simulink model "simulation"  (R2013b)
settings: Solver=ode45  StartTime=0.0  StopTime=2000  RelTol=1e-3
values from neighbouring files (symbols this model uses):
  delta = .5    (= 0.5)    [simulation_init.m]
  Fmax = 1000    [simulation_init.m]
  Fmin = -750    [simulation_init.m]
  J = I_z - N    (= 2752.5)    [simulation_init.m]
  k_r = .5    (= 0.5)    [simulation_init.m]
  k_u = .5    (= 0.5)    [simulation_init.m]
  k_xi = 1    [simulation_init.m]
  kx = .3    (= 0.3)    [simulation_init.m]
  ky = .15    (= 0.15)    [simulation_init.m]
  kz = 1.5    [simulation_init.m]
  l = 1    [simulation_init.m]
  m_u = m - Xm_u    (= 4287.13636)    [simulation_init.m]
  m_uv = Xm_v - Xm_u    (= -28.713636)    [simulation_init.m]
  m_v = m - Xm_v    (= 4315.849996)    [simulation_init.m]
  n = 4    [simulation_init.m]
  noiseon = 1    [simulation_init.m]
  npsi = 0.00005    (= 5e-05)    [simulation_init.m]
  npsi_c = 0*.00005    (= 0)    [simulation_init.m]
  Nr = -110    [simulation_init.m]
  nr = 0.005    [simulation_init.m]
  Nrr = -555    [simulation_init.m]
  nsonar = .1    (= 0.1)    [simulation_init.m]
  nu = .05    (= 0.05)    [simulation_init.m]
  nv = 0.005    [simulation_init.m]
  nVc = 0*.005    (= 0)    [simulation_init.m]
  P01 = [20   20]    [simulation_init.m]
  P02 = [40   00]    [simulation_init.m]
  P03 = [20  -20]    [simulation_init.m]
  P04 = [150 40]    [simulation_init.m]
  psi01 = 0*pi/180    (= 0)    [simulation_init.m]
  psi02 = 0*pi/180    (= 0)    [simulation_init.m]
  psi03 = 0*pi/180    (= 0)    [simulation_init.m]
  psi_c = 45*pi/180    (= 0.785398163397)    [simulation_init.m]
  Q1 = diag([nu nv npsi])    [simulation_init.m]
  Q2 = diag([nu nv npsi])    [simulation_init.m]
  Q3 = diag([nu nv npsi])    [simulation_init.m]
  Sigma01 = 15*eye(3)    [simulation_init.m]
  Sigma02 = Sigma01    [simulation_init.m]
  Sigma03 = Sigma01    [simulation_init.m]
  State_est01 = [P01+[sN(1),sN(2)] psi01]    [simulation_init.m]
  State_est02 = [P02+[sN(3),sN(4)] psi02]    [simulation_init.m]
  State_est03 = [P03+[sN(5),sN(6)] psi03]    [simulation_init.m]
  T_bc = 1    [simulation_init.m]
  T_est = .1    (= 0.1)    [simulation_init.m]
  Vc = .3    (= 0.3)    [simulation_init.m]
  Xu = -360    [simulation_init.m]
  Xuu = -805    [simulation_init.m]
  Yv = -420    [simulation_init.m]
  Yvv = -1930    [simulation_init.m]
undefined symbols (not defined in the file or in its folder): Pathdata
libraries: simulink x22
(part 1 of 2)
settings Model: Creator=Andreas  LastModifiedBy=Andreas

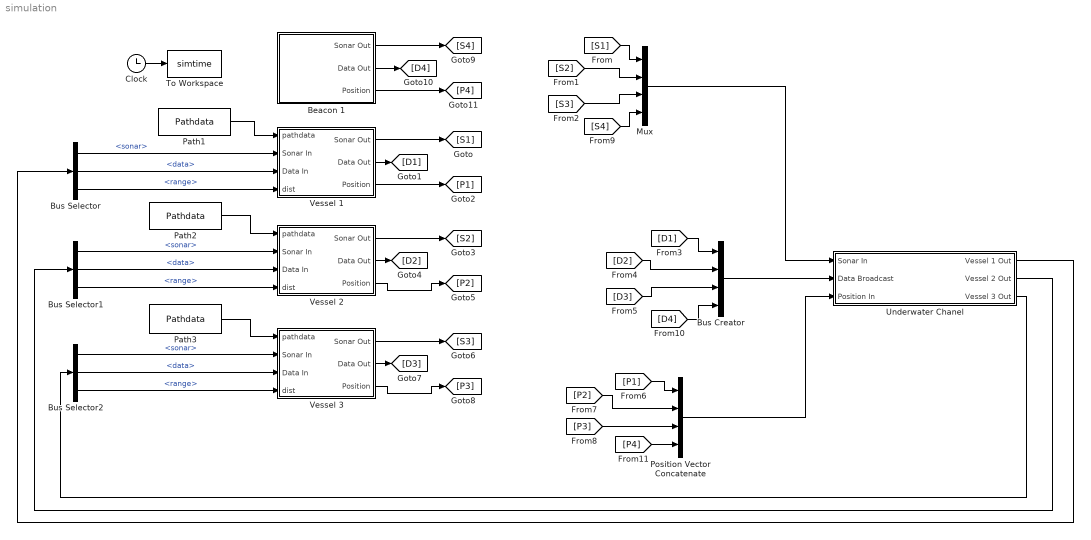
== system simulation ==
  Beacon 1 : Subsystem  mask{i=4}
      mask prompts: i "id"
  Bus Creator : BusCreator
  Bus Selector : BusSelector  OutputSignals=sonar,data,range
  Bus Selector1 : BusSelector  OutputSignals=sonar,data,range
  Bus Selector2 : BusSelector  OutputSignals=sonar,data,range
  Clock : Clock
  Mux : Mux
  Path1 : Constant  Value=Pathdata
  Path2 : Constant  Value=Pathdata
  Path3 : Constant  Value=Pathdata
  Position Vector Concatenate : Concatenate  NumInputs=4  Mode=Multidimensional array  ConcatenateDimension=2
  To Workspace : ToWorkspace  VariableName=simtime  SampleTime=-1
  Underwater Chanel : Subsystem
  Vessel 1 : Subsystem  mask{i=1}
      mask prompts: i "id"
      mask init:
      | Maskinit
  Vessel 2 : Subsystem  mask{i=2}
      mask prompts: i "id"
      mask init:
      | Maskinit
  Vessel 3 : Subsystem  mask{i=3}
      mask prompts: i "id"
      mask init:
      | Maskinit
  wires:
  Underwater Chanel/1(Vessel 1 Out) -> Bus Selector/1
  Underwater Chanel/2(Vessel 2 Out) -> Bus Selector1/1
  Underwater Chanel/3(Vessel 3 Out) -> Bus Selector2/1
  [S1] -> Mux/1
  [S3] -> Mux/3
  [D1] -> Bus Creator/1
  [D2] -> Bus Creator/2
  [D3] -> Bus Creator/3
  [P2] -> Position Vector Concatenate/2
  [P1] -> Position Vector Concatenate/1
  [P3] -> Position Vector Concatenate/3
  Vessel 1/1(Sonar Out) -> [S1]
  Vessel 1/2(Data Out) -> [D1]
  Vessel 1/3(Position) -> [P1]
  Vessel 2/1(Sonar Out) -> [S2]
  Vessel 2/2(Data Out) -> [D2]
  Vessel 2/3(Position) -> [P2]
  Vessel 3/1(Sonar Out) -> [S3]
  Vessel 3/2(Data Out) -> [D3]
  Vessel 3/3(Position) -> [P3]
  Position Vector Concatenate/1 -> Underwater Chanel/3(Position In)
  [S2] -> Mux/2
  Path1/1 -> Vessel 1/1(pathdata)
  Path2/1 -> Vessel 2/1(pathdata)
  Path3/1 -> Vessel 3/1(pathdata)
  Clock/1 -> To Workspace/1
  Beacon 1/1(Sonar Out) -> [S4]
  Beacon 1/2(Data Out) -> [D4]
  Beacon 1/3(Position) -> [P4]
  [S4] -> Mux/4
  [D4] -> Bus Creator/4
  [P4] -> Position Vector Concatenate/4
  Bus Selector/2 -> Vessel 1/3(Data In)  "<data>"
  Bus Selector/1 -> Vessel 1/2(Sonar In)  "<sonar>"
  Bus Selector/3 -> Vessel 1/4(dist)  "<range>"
  Bus Selector2/1 -> Vessel 3/2(Sonar In)  "<sonar>"
  Bus Selector2/3 -> Vessel 3/4(dist)  "<range>"
  Bus Selector2/2 -> Vessel 3/3(Data In)  "<data>"
  Bus Selector1/3 -> Vessel 2/4(dist)  "<range>"
  Bus Selector1/2 -> Vessel 2/3(Data In)  "<data>"
  Bus Selector1/1 -> Vessel 2/2(Sonar In)  "<sonar>"
  Mux/1 -> Underwater Chanel/1(Sonar In)
  Bus Creator/1 -> Underwater Chanel/2(Data Broadcast)

== system simulation/Beacon 1 ==
  Constant : Constant
  Cov : Constant  Value=0.0001*[1 0 0 1]
  Fixed Position : Constant  Value=[P04 0]
  Fixed Position2 : Constant  Value=P04
  JLaw : simulink/Sources/Repeating Sequence Stair  OutValues=TrsmtLaw.'  tsamp=T_bc  OutMin=[]  OutMax=[]  OutDataTypeStr=double  OutputDataTypeScalingMode=double  OutDataType=fixdt(0,8)  ConRadixGroup=Best Precision: Vector-wise  OutScaling=2^-12
  Transmitter : Subsystem
  data_out : ToWorkspace  VariableName=data_out4  SampleTime=-1
  sonar_out : ToWorkspace  VariableName=sonar_out4  SampleTime=-1
  Sonar Out : Outport
  Data Out : Outport  Port=2
  Position : Outport  Port=3
  wires:
  Constant/1 -> Transmitter/3(gamma_i1)
  JLaw/1 -> Transmitter/1(j1)
  Fixed Position/1 -> Position/1
  Transmitter/1(Sonar Out) -> sonar_out/1, Sonar Out/1
  Transmitter/2(Data Out) -> Data Out/1, data_out/1
  Cov/1 -> Transmitter/4(cov1)
  Fixed Position2/1 -> Transmitter/2(state1)

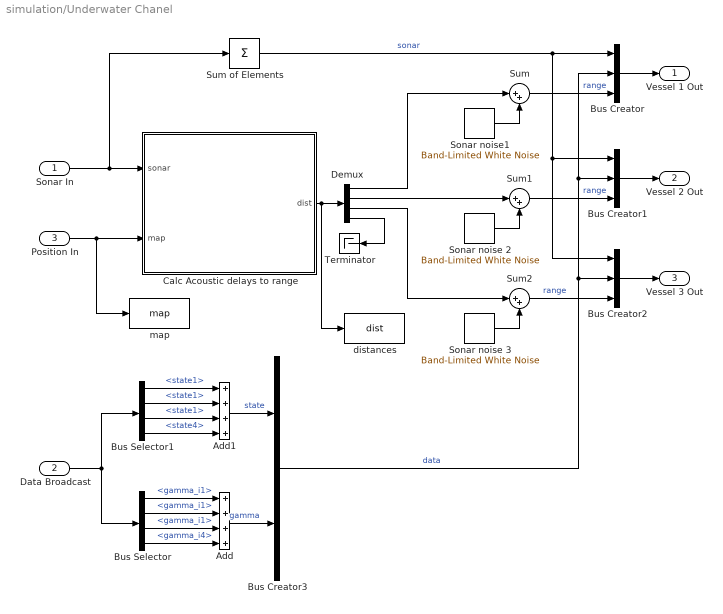
== system simulation/Underwater Chanel ==
  Sonar In : Inport
  Data Broadcast : Inport  Port=2
  Position In : Inport  Port=3
  Add : Sum  Inputs=++++
  Add1 : Sum  Inputs=++++
  Bus Creator : BusCreator  Inputs=3
  Bus Creator1 : BusCreator  Inputs=3
  Bus Creator2 : BusCreator  Inputs=3
  Bus Creator3 : BusCreator  Inputs=2
  Bus Selector : BusSelector  OutputSignals=signal1.gamma_i1,signal2.gamma_i1,signal3.gamma_i1,signal4.gamma_i4
  Bus Selector1 : BusSelector  OutputSignals=signal1.state1,signal2.state1,signal3.state1,signal4.state4
  Calc Acoustic delays to range : MATLAB Function  TreatAsAtomicUnit=on
  Demux : Demux
  Sonar noise 2 : simulink/Sources/Band-Limited White Noise  Cov=noiseon*nsonar*0.1  Ts=0.1  seed=535
  Sonar noise 3 : simulink/Sources/Band-Limited White Noise  Cov=noiseon*nsonar*0.1  Ts=0.1  seed=24
  Sonar noise1 : simulink/Sources/Band-Limited White Noise  Cov=noiseon*nsonar*0.1  Ts=0.1  seed=[253]
  Sum : Sum  Inputs=|++
  Sum of Elements : Sum  Inputs=+
  Sum1 : Sum  Inputs=|++
  Sum2 : Sum  Inputs=|++
  Terminator : Terminator
  distances : ToWorkspace  VariableName=dist  SampleTime=-1
  map : ToWorkspace  VariableName=map  SampleTime=-1
  Vessel 1 Out : Outport
  Vessel 2 Out : Outport  Port=2
  Vessel 3 Out : Outport  Port=3
  wires:
  Position In/1 -> map/1, Calc Acoustic delays to range/2(map)
  Bus Creator/1 -> Vessel 1 Out/1
  Bus Creator2/1 -> Vessel 3 Out/1
  Calc Acoustic delays to range/1(dist) -> distances/1, Demux/1
  Sonar In/1 -> Sum of Elements/1, Calc Acoustic delays to range/1(sonar)
  Bus Creator1/1 -> Vessel 2 Out/1
  Data Broadcast/1 -> Bus Selector1/1, Bus Selector/1
  Sum of Elements/1 -> Bus Creator/1, Bus Creator2/1, Bus Creator1/1  "sonar"
  Demux/4 -> Terminator/1
  Sum/1 -> Bus Creator/3  "range"
  Demux/1 -> Sum/1
  Sonar noise1/1 -> Sum/2
  Sonar noise 2/1 -> Sum1/2
  Demux/2 -> Sum1/1
  Sum1/1 -> Bus Creator1/3  "range"
  Sonar noise 3/1 -> Sum2/2
  Demux/3 -> Sum2/1
  Sum2/1 -> Bus Creator2/3  "range"
  Bus Selector/2 -> Add/2  "<gamma_i1>"
  Bus Selector/1 -> Add/1  "<gamma_i1>"
  Bus Selector/3 -> Add/3  "<gamma_i1>"
  Bus Selector1/3 -> Add1/3  "<state1>"
  Bus Selector1/1 -> Add1/1  "<state1>"
  Bus Selector1/4 -> Add1/4  "<state4>"
  Bus Selector1/2 -> Add1/2  "<state1>"
  Add1/1 -> Bus Creator3/1  "state"
  Add/1 -> Bus Creator3/2  "gamma"
  Bus Creator3/1 -> Bus Creator2/2, Bus Creator1/2, Bus Creator/2  "data"
  Bus Selector/4 -> Add/4  "<gamma_i4>"

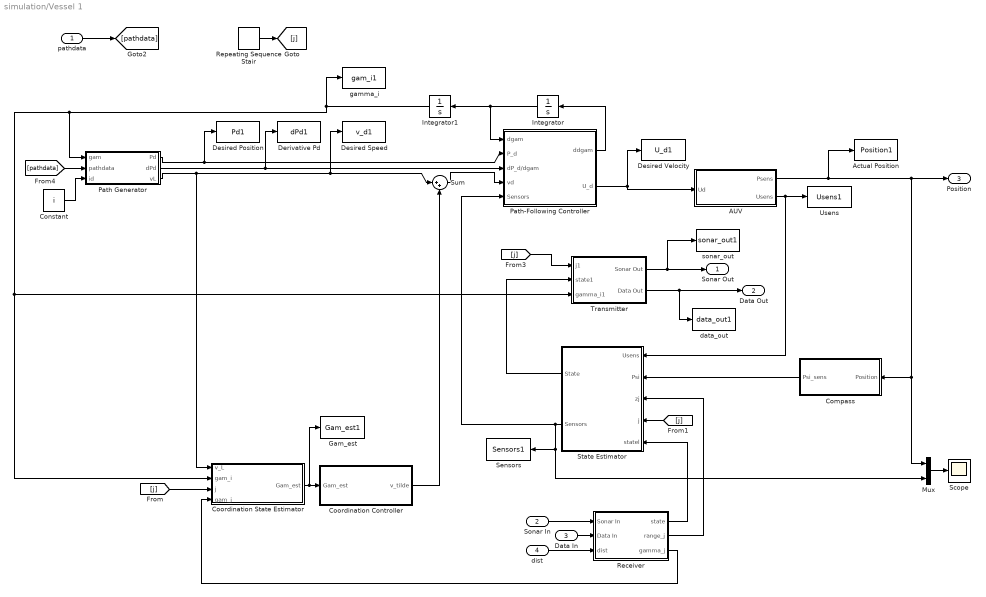
== system simulation/Vessel 1 ==
  pathdata : Inport
  Sonar In : Inport  Port=2
  Data In : Inport  Port=3
  dist : Inport  Port=4
  AUV : Subsystem
  Actual Position : ToWorkspace  VariableName=Position1  SampleTime=-1
  Compass : Subsystem
  Constant : Constant  Value=i
  Coordination Controller : MATLAB Function  TreatAsAtomicUnit=on
  Coordination State Estimator : Subsystem
  Derivative Pd : ToWorkspace  VariableName=dPd1  SampleTime=-1
  Desired Position : ToWorkspace  VariableName=Pd1  SampleTime=-1
  Desired Speed : ToWorkspace  VariableName=v_d1  SampleTime=-1
  Desired Velocity : ToWorkspace  VariableName=U_d1  SampleTime=-1
  Gam_est : ToWorkspace  VariableName=Gam_est1  SampleTime=-1
  Integrator : Integrator
  Integrator1 : Integrator
  Mux : Mux  Inputs=2
  Path Generator : Subsystem
  Path-Following Controller : Subsystem
  Receiver : Subsystem
  Repeating Sequence Stair : simulink/Sources/Repeating Sequence Stair  OutValues=TrsmtLaw.'  tsamp=T_bc  OutMin=[]  OutMax=[]  OutDataTypeStr=double  OutputDataTypeScalingMode=double  OutDataType=fixdt(0,8)  ConRadixGroup=Best Precision: Vector-wise  OutScaling=2^-12
  Scope : Scope
      settings: YMin=-25  YMax=275
  Sensors : ToWorkspace  VariableName=Sensors1  SampleTime=-1
  State Estimator : Subsystem
  Sum : Sum  Inputs=|++
  Transmitter : Subsystem
  Usens : ToWorkspace  VariableName=Usens1  SampleTime=-1
  data_out : ToWorkspace  VariableName=data_out1  SampleTime=-1
  gamma_i : ToWorkspace  VariableName=gam_i1  SampleTime=-1
  sonar_out : ToWorkspace  VariableName=sonar_out1  SampleTime=-1
  Sonar Out : Outport
  Data Out : Outport  Port=2
  Position : Outport  Port=3
  wires:
  Sonar In/1 -> Receiver/1(Sonar In)
  Data In/1 -> Receiver/2(Data In)
  Integrator1/1 -> gamma_i/1, Path Generator/1(gam), Transmitter/3(gamma_i1), Coordination State Estimator/2(gam_i)
  Path Generator/3(vL) -> Coordination State Estimator/1(v_L), Desired Speed/1, Sum/1
  Coordination Controller/1(v_tilde) -> Sum/2
  Sum/1 -> Path-Following Controller/4(vd)
  Transmitter/1(Sonar Out) -> sonar_out/1, Sonar Out/1
  Transmitter/2(Data Out) -> data_out/1, Data Out/1
  Receiver/3(gamma_j) -> Coordination State Estimator/4(gam_j)
  Path Generator/1(Pd) -> Desired Position/1, Path-Following Controller/2(P_d)
  Path-Following Controller/1(ddgam) -> Integrator/1
  Integrator/1 -> Integrator1/1, Path-Following Controller/1(dgam)
  Path-Following Controller/2(U_d) -> AUV/1(Ud), Desired Velocity/1
  AUV/2(Usens) -> Usens/1, State Estimator/1(Usens)
  AUV/1(Psens) -> Mux/1, Compass/1(Position), Position/1, Actual Position/1
  Coordination State Estimator/1(Gam_est) -> Gam_est/1, Coordination Controller/1(Gam_est)
  Path Generator/2(dPd) -> Path-Following Controller/3(dP_d/dgam), Derivative Pd/1
  Repeating Sequence Stair/1 -> [j]
  [j] -> Coordination State Estimator/3(j)
  dist/1 -> Receiver/3(dist)
  Constant/1 -> Path Generator/3(id)
  pathdata/1 -> [pathdata]
  [pathdata] -> Path Generator/2(pathdata)
  State Estimator/2(Sensors) -> Sensors/1, Mux/2, Path-Following Controller/5(Sensors)
  [j] -> Transmitter/1(j1)
  [j] -> State Estimator/4(j)
  State Estimator/1("State ") -> Transmitter/2(state1)
  Receiver/1(state) -> State Estimator/5(statel)
  Mux/1 -> Scope/1
  Compass/1(Psi_sens) -> State Estimator/2(Psi)
  Receiver/2(range_j) -> State Estimator/3(zj)

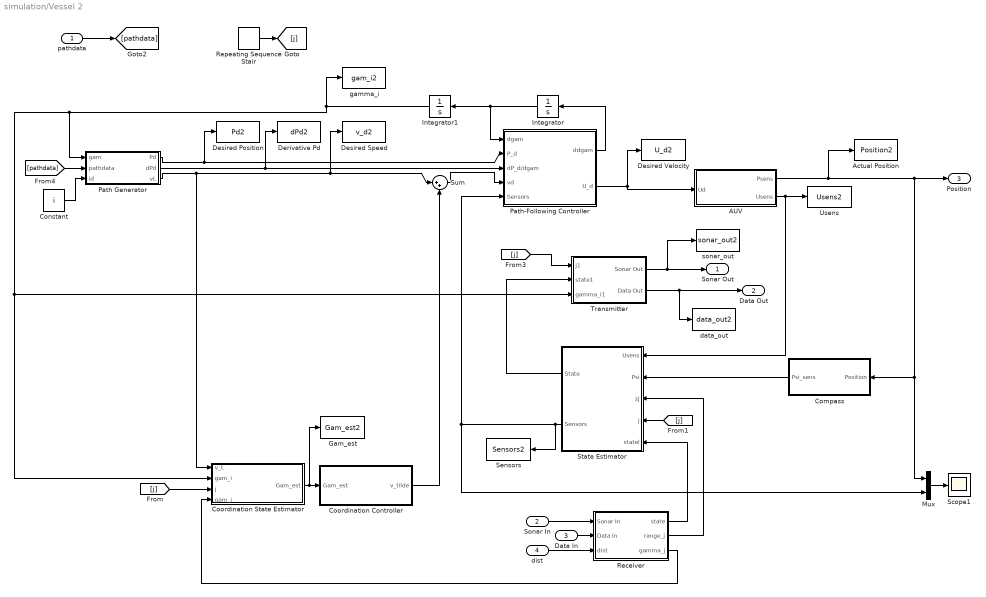
== system simulation/Vessel 2 ==
  pathdata : Inport
  Sonar In : Inport  Port=2
  Data In : Inport  Port=3
  dist : Inport  Port=4
  AUV : Subsystem
  Actual Position : ToWorkspace  VariableName=Position2  SampleTime=-1
  Compass : Subsystem
  Constant : Constant  Value=i
  Coordination Controller : MATLAB Function  TreatAsAtomicUnit=on
  Coordination State Estimator : Subsystem
  Derivative Pd : ToWorkspace  VariableName=dPd2  SampleTime=-1
  Desired Position : ToWorkspace  VariableName=Pd2  SampleTime=-1
  Desired Speed : ToWorkspace  VariableName=v_d2  SampleTime=-1
  Desired Velocity : ToWorkspace  VariableName=U_d2  SampleTime=-1
  Gam_est : ToWorkspace  VariableName=Gam_est2  SampleTime=-1
  Integrator : Integrator
  Integrator1 : Integrator
  Mux : Mux  Inputs=2
  Path Generator : Subsystem
  Path-Following Controller : Subsystem
  Receiver : Subsystem
  Repeating Sequence Stair : simulink/Sources/Repeating Sequence Stair  OutValues=TrsmtLaw.'  tsamp=T_bc  OutMin=[]  OutMax=[]  OutDataTypeStr=double  OutputDataTypeScalingMode=double  OutDataType=fixdt(0,8)  ConRadixGroup=Best Precision: Vector-wise  OutScaling=2^-12
  Scope1 : Scope
      settings: YMin=-25  YMax=275
  Sensors : ToWorkspace  VariableName=Sensors2  SampleTime=-1
  State Estimator : Subsystem
  Sum : Sum  Inputs=|++
  Transmitter : Subsystem
  Usens : ToWorkspace  VariableName=Usens2  SampleTime=-1
  data_out : ToWorkspace  VariableName=data_out2  SampleTime=-1
  gamma_i : ToWorkspace  VariableName=gam_i2  SampleTime=-1
  sonar_out : ToWorkspace  VariableName=sonar_out2  SampleTime=-1
  Sonar Out : Outport
  Data Out : Outport  Port=2
  Position : Outport  Port=3
  wires:
  Receiver/1(state) -> State Estimator/5(statel)
  State Estimator/1("State ") -> Transmitter/2(state1)
  [j] -> State Estimator/4(j)
  [j] -> Transmitter/1(j1)
  [pathdata] -> Path Generator/2(pathdata)
  pathdata/1 -> [pathdata]
  Constant/1 -> Path Generator/3(id)
  dist/1 -> Receiver/3(dist)
  [j] -> Coordination State Estimator/3(j)
  Repeating Sequence Stair/1 -> [j]
  Path Generator/2(dPd) -> Derivative Pd/1, Path-Following Controller/3(dP_d/dgam)
  Coordination State Estimator/1(Gam_est) -> Coordination Controller/1(Gam_est), Gam_est/1
  AUV/2(Usens) -> State Estimator/1(Usens), Usens/1
  Path-Following Controller/2(U_d) -> Desired Velocity/1, AUV/1(Ud)
  Integrator/1 -> Path-Following Controller/1(dgam), Integrator1/1
  Path-Following Controller/1(ddgam) -> Integrator/1
  Path Generator/1(Pd) -> Path-Following Controller/2(P_d), Desired Position/1
  Receiver/3(gamma_j) -> Coordination State Estimator/4(gam_j)
  Transmitter/2(Data Out) -> Data Out/1, data_out/1
  Transmitter/1(Sonar Out) -> Sonar Out/1, sonar_out/1
  Sum/1 -> Path-Following Controller/4(vd)
  Coordination Controller/1(v_tilde) -> Sum/2
  Path Generator/3(vL) -> Sum/1, Desired Speed/1, Coordination State Estimator/1(v_L)
  Integrator1/1 -> Coordination State Estimator/2(gam_i), Transmitter/3(gamma_i1), Path Generator/1(gam), gamma_i/1
  Data In/1 -> Receiver/2(Data In)
  Sonar In/1 -> Receiver/1(Sonar In)
  AUV/1(Psens) -> Actual Position/1, Compass/1(Position), Mux/1, Position/1
  State Estimator/2(Sensors) -> Path-Following Controller/5(Sensors), Mux/2, Sensors/1
  Mux/1 -> Scope1/1
  Compass/1(Psi_sens) -> State Estimator/2(Psi)
  Receiver/2(range_j) -> State Estimator/3(zj)

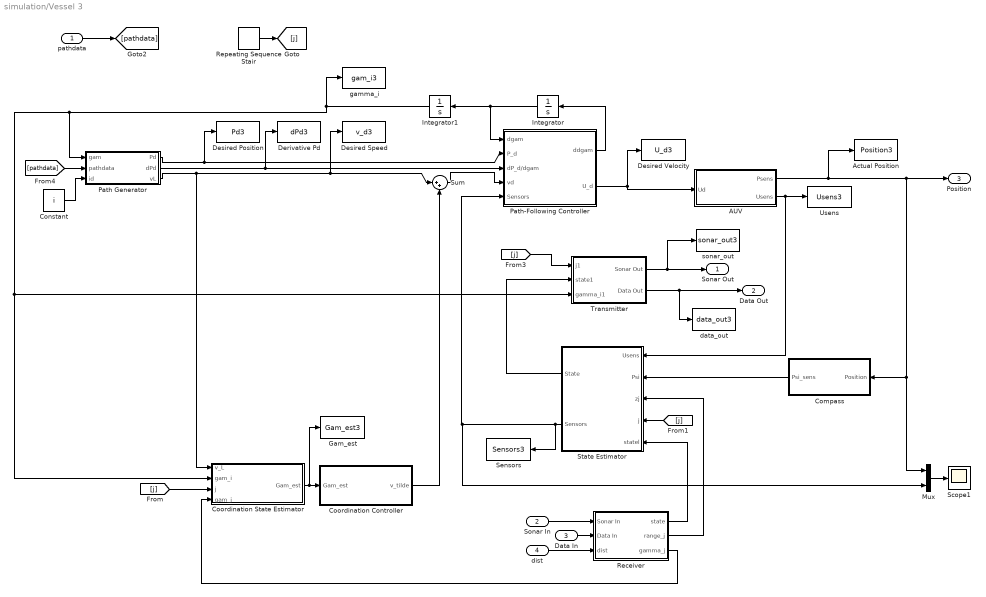
== system simulation/Vessel 3 ==
  pathdata : Inport
  Sonar In : Inport  Port=2
  Data In : Inport  Port=3
  dist : Inport  Port=4
  AUV : Subsystem
  Actual Position : ToWorkspace  VariableName=Position3  SampleTime=-1
  Compass : Subsystem
  Constant : Constant  Value=i
  Coordination Controller : MATLAB Function  TreatAsAtomicUnit=on
  Coordination State Estimator : Subsystem
  Derivative Pd : ToWorkspace  VariableName=dPd3  SampleTime=-1
  Desired Position : ToWorkspace  VariableName=Pd3  SampleTime=-1
  Desired Speed : ToWorkspace  VariableName=v_d3  SampleTime=-1
  Desired Velocity : ToWorkspace  VariableName=U_d3  SampleTime=-1
  Gam_est : ToWorkspace  VariableName=Gam_est3  SampleTime=-1
  Integrator : Integrator
  Integrator1 : Integrator
  Mux : Mux  Inputs=2
  Path Generator : Subsystem
  Path-Following Controller : Subsystem
  Receiver : Subsystem
  Repeating Sequence Stair : simulink/Sources/Repeating Sequence Stair  OutValues=TrsmtLaw.'  tsamp=T_bc  OutMin=[]  OutMax=[]  OutDataTypeStr=double  OutputDataTypeScalingMode=double  OutDataType=fixdt(0,8)  ConRadixGroup=Best Precision: Vector-wise  OutScaling=2^-12
  Scope1 : Scope
      settings: YMin=-10  YMax=130  SaveName=ScopeData2
  Sensors : ToWorkspace  VariableName=Sensors3  SampleTime=-1
  State Estimator : Subsystem
  Sum : Sum  Inputs=|++
  Transmitter : Subsystem
  Usens : ToWorkspace  VariableName=Usens3  SampleTime=-1
  data_out : ToWorkspace  VariableName=data_out3  SampleTime=-1
  gamma_i : ToWorkspace  VariableName=gam_i3  SampleTime=-1
  sonar_out : ToWorkspace  VariableName=sonar_out3  SampleTime=-1
  Sonar Out : Outport
  Data Out : Outport  Port=2
  Position : Outport  Port=3
  wires:
  Sonar In/1 -> Receiver/1(Sonar In)
  Data In/1 -> Receiver/2(Data In)
  Integrator1/1 -> gamma_i/1, Path Generator/1(gam), Transmitter/3(gamma_i1), Coordination State Estimator/2(gam_i)
  Path Generator/3(vL) -> Coordination State Estimator/1(v_L), Desired Speed/1, Sum/1
  Coordination Controller/1(v_tilde) -> Sum/2
  Sum/1 -> Path-Following Controller/4(vd)
  Transmitter/1(Sonar Out) -> sonar_out/1, Sonar Out/1
  Transmitter/2(Data Out) -> data_out/1, Data Out/1
  Receiver/3(gamma_j) -> Coordination State Estimator/4(gam_j)
  Path Generator/1(Pd) -> Desired Position/1, Path-Following Controller/2(P_d)
  Path-Following Controller/1(ddgam) -> Integrator/1
  Integrator/1 -> Integrator1/1, Path-Following Controller/1(dgam)
  Path-Following Controller/2(U_d) -> AUV/1(Ud), Desired Velocity/1
  AUV/2(Usens) -> Usens/1, State Estimator/1(Usens)
  Coordination State Estimator/1(Gam_est) -> Gam_est/1, Coordination Controller/1(Gam_est)
  Path Generator/2(dPd) -> Path-Following Controller/3(dP_d/dgam), Derivative Pd/1
  Repeating Sequence Stair/1 -> [j]
  [j] -> Coordination State Estimator/3(j)
  dist/1 -> Receiver/3(dist)
  Constant/1 -> Path Generator/3(id)
  pathdata/1 -> [pathdata]
  [pathdata] -> Path Generator/2(pathdata)
  [j] -> Transmitter/1(j1)
  [j] -> State Estimator/4(j)
  State Estimator/1("State ") -> Transmitter/2(state1)
  Receiver/1(state) -> State Estimator/5(statel)
  AUV/1(Psens) -> Position/1, Compass/1(Position), Mux/1, Actual Position/1
  State Estimator/2(Sensors) -> Sensors/1, Path-Following Controller/5(Sensors), Mux/2
  Mux/1 -> Scope1/1
  Compass/1(Psi_sens) -> State Estimator/2(Psi)
  Receiver/2(range_j) -> State Estimator/3(zj)

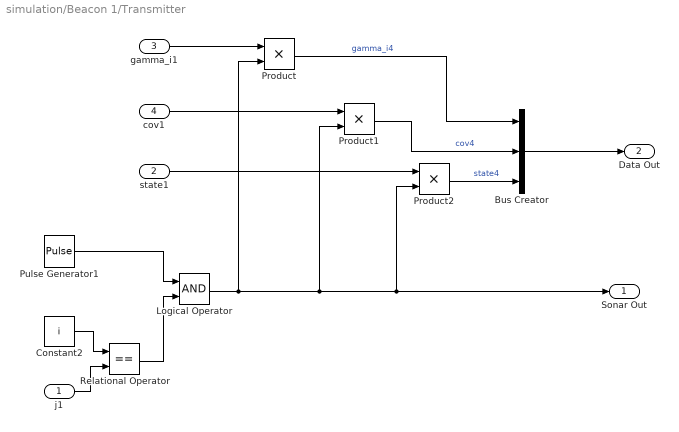
== system simulation/Beacon 1/Transmitter ==
  j1 : Inport
  state1 : Inport  Port=2
  gamma_i1 : Inport  Port=3
  cov1 : Inport  Port=4
  Bus Creator : BusCreator  Inputs=3
  Constant2 : Constant  Value=i
  Logical Operator : Logic  AllPortsSameDT=off  OutDataTypeStr=boolean
  Product : Product
  Product1 : Product
  Product2 : Product
  Pulse Generator1 : DiscretePulseGenerator  PulseType=Time based  Period=T_bc  PulseWidth=.001/( T_bc)*100
  Relational Operator : RelationalOperator  Operator===  OutDataTypeStr=boolean
  Sonar Out : Outport
  Data Out : Outport  Port=2
  wires:
  Pulse Generator1/1 -> Logical Operator/1
  j1/1 -> Relational Operator/2
  Constant2/1 -> Relational Operator/1
  Relational Operator/1 -> Logical Operator/2
  Logical Operator/1 -> Product/2, Product1/2, Product2/2, Sonar Out/1
  Bus Creator/1 -> Data Out/1
  gamma_i1/1 -> Product/1
  cov1/1 -> Product1/1
  state1/1 -> Product2/1
  Product/1 -> Bus Creator/1  "gamma_i4"
  Product1/1 -> Bus Creator/2  "cov4"
  Product2/1 -> Bus Creator/3  "state4"

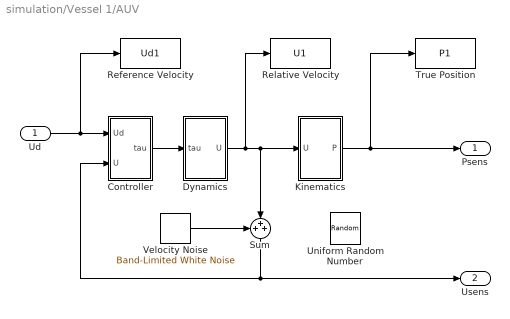
== system simulation/Vessel 1/AUV ==
  Ud : Inport
  Controller : Subsystem
  Dynamics : Subsystem
  Kinematics : Subsystem
  Reference Velocity : ToWorkspace  VariableName=Ud1  SampleTime=-1
  Relative Velocity : ToWorkspace  VariableName=U1  SampleTime=-1
  Sum : Sum  Inputs=+++
  True Position : ToWorkspace  VariableName=P1  SampleTime=-1
  Uniform Random Number : UniformRandomNumber  Minimum=-5*noiseon*[nu nv nr]  Maximum=5*noiseon*[nu nv nr]  Seed=[1627 9317 3723]  SampleTime=20
  Velocity Noise : simulink/Sources/Band-Limited White Noise  Cov=noiseon*[nu nv nr]*0.1  Ts=0.1  seed=[2334 8715 567]
  Psens : Outport
  Usens : Outport  Port=2
  wires:
  Dynamics/1(U) -> Relative Velocity/1, Sum/2, Kinematics/1(U)
  Controller/1(tau) -> Dynamics/1(tau)
  Ud/1 -> Controller/1(Ud), Reference Velocity/1
  Velocity Noise/1 -> Sum/1
  Sum/1 -> Controller/2(U), Usens/1
  Kinematics/1(P) -> Psens/1, True Position/1

== system simulation/Vessel 1/Compass ==
  Position : Inport
  Compass noise : simulink/Sources/Band-Limited White Noise  Cov=noiseon*npsi*0.1  Ts=0.1  seed=9167
  Demux : Demux  Outputs=3
  Mux1 : Mux  Inputs=2
  Sum : Sum  Inputs=|++
  Sum1 : Sum  Inputs=+|+
  Terminator1 : Terminator
  calibration error : simulink/Sources/Band-Limited White Noise  Cov=noiseon*npsi*200  Ts=200  seed=7691
  Psi_sens : Outport
  wires:
  Demux/2 -> Mux1/2
  Mux1/1 -> Terminator1/1
  Demux/1 -> Mux1/1
  Sum/1 -> Psi_sens/1
  Demux/3 -> Sum/1
  Position/1 -> Demux/1
  Sum1/1 -> Sum/2
  Compass noise/1 -> Sum1/1
  calibration error/1 -> Sum1/2

== system simulation/Vessel 1/Coordination State Estimator ==
  v_L : Inport
  gam_i : Inport  Port=2
  j : Inport  Port=3
  gam_j : Inport  Port=4
  Integrator2 : Integrator  InitialCondition=zeros(1,n)
  "Update " : MATLAB Function  TreatAsAtomicUnit=on
  Gam_est : Outport
  wires:
  v_L/1 -> Integrator2/1
  Integrator2/1 -> "Update "/1(Gam_predict)
  gam_i/1 -> "Update "/2(gam_i)
  gam_j/1 -> "Update "/3(gam_j)
  j/1 -> "Update "/4(j)
  "Update "/1(Gam_est) -> Gam_est/1

== system simulation/Vessel 1/Path Generator ==
  gam : Inport
  pathdata : Inport  Port=2
  id : Inport  Port=3
  Nominal Values Generator : Subsystem
  Read Pathdata : Subsystem
  Pd : Outport
  dPd : Outport  Port=2
  vL : Outport  Port=3
  wires:
  Nominal Values Generator/3(v_L) -> vL/1
  Nominal Values Generator/2(dP_d) -> dPd/1
  Nominal Values Generator/1(P_d) -> Pd/1
  gam/1 -> Nominal Values Generator/1(gam), Read Pathdata/1(gam)
  pathdata/1 -> Read Pathdata/2(pathdata)
  id/1 -> Read Pathdata/3(id)
  Read Pathdata/1(path params) -> Nominal Values Generator/2(path params)

== system simulation/Vessel 1/Path-Following Controller ==
  dgam : Inport
  P_d : Inport  Port=2
  dP_d/dgam : Inport  Port=3
  vd : Inport  Port=4
  Sensors : Inport  Port=5
  Demux : Demux  Outputs=3
  PF Control Law : MATLAB Function  TreatAsAtomicUnit=on
  Path following error : ToWorkspace  VariableName=PFerror1  SampleTime=-1
  ddgam : Outport
  U_d : Outport  Port=2
  wires:
  Sensors/1 -> Demux/1
  vd/1 -> PF Control Law/6(Vd)
  dP_d/dgam/1 -> PF Control Law/5(dPd)
  P_d/1 -> PF Control Law/4(Pd)
  dgam/1 -> PF Control Law/7(dgam)
  PF Control Law/1(Ud) -> U_d/1
  PF Control Law/3(ddgam) -> ddgam/1
  Demux/1 -> PF Control Law/1(Vc)
  Demux/3 -> PF Control Law/3(psi)
  Demux/2 -> PF Control Law/2(P)
  PF Control Law/2(e) -> Path following error/1

== system simulation/Vessel 1/Receiver ==
  Sonar In : Inport
  Data In : Inport  Port=2
  dist : Inport  Port=3
  Bus Selector : BusSelector  OutputSignals=gamma,state
  Terminator : Terminator
  state : Outport
  range_j : Outport  Port=2
  gamma_j : Outport  Port=3
  wires:
  Sonar In/1 -> Terminator/1
  Data In/1 -> Bus Selector/1
  dist/1 -> range_j/1
  Bus Selector/1 -> gamma_j/1  "<gamma>"
  Bus Selector/2 -> state/1  "<state>"

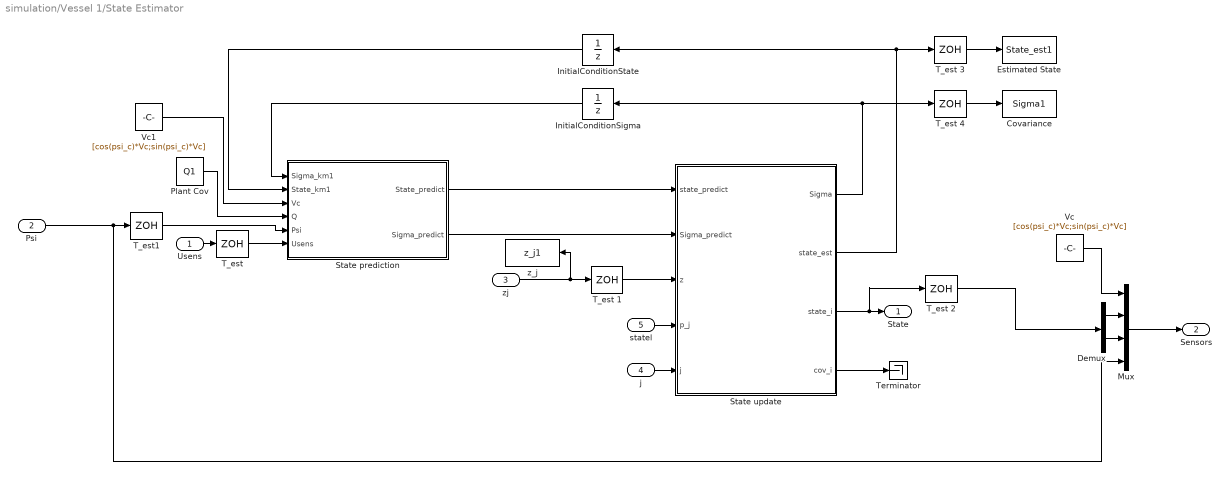
== system simulation/Vessel 1/State Estimator ==
  Usens : Inport
  Psi : Inport  Port=2
  zj : Inport  Port=3
  j : Inport  Port=4
  statel : Inport  Port=5
  Covariance : ToWorkspace  VariableName=Sigma1  SampleTime=-1
  Demux : Demux  Outputs=2
  Estimated State : ToWorkspace  VariableName=State_est1  SampleTime=-1
  InitialConditionSigma : UnitDelay  InitialCondition=Sigma01  SampleTime=T_est
  InitialConditionState : UnitDelay  InitialCondition=State_est01  SampleTime=T_est
  Mux : Mux
  Plant Cov : Constant  Value=Q1
  State prediction : MATLAB Function  TreatAsAtomicUnit=on
  State update : MATLAB Function  TreatAsAtomicUnit=on
  T_est {,1..4} (5 alike) : ZeroOrderHold  SampleTime=T_est
  "T_est1 " : ZeroOrderHold  SampleTime=T_est
  Terminator : Terminator
  Vc : Constant  Value=[cos(psi_c)*Vc;sin(psi_c)*Vc]
  Vc1 : Constant  Value=[cos(psi_c)*Vc;sin(psi_c)*Vc]
  z_j : ToWorkspace  VariableName=z_j1  SampleTime=-1
  "State " : Outport
  Sensors : Outport  Port=2
  wires:
  State prediction/1(State_predict) -> State update/1(state_predict)
  State update/2(state_est) -> T_est 3/1, InitialConditionState/1
  State prediction/2(Sigma_predict) -> State update/2(Sigma_predict)
  State update/1(Sigma) -> T_est 4/1, InitialConditionSigma/1
  InitialConditionSigma/1 -> State prediction/1(Sigma_km1)
  InitialConditionState/1 -> State prediction/2(State_km1)
  Usens/1 -> "T_est "/1
  Mux/1 -> Sensors/1
  Vc/1 -> Mux/1
  Psi/1 -> Mux/4, "T_est1 "/1
  Plant Cov/1 -> State prediction/4(Q)
  zj/1 -> T_est 1/1, z_j/1
  "T_est1 "/1 -> State prediction/5(Psi)
  "T_est "/1 -> State prediction/6(Usens)
  Vc1/1 -> State prediction/3(Vc)
  j/1 -> State update/5(j)
  State update/3(state_i) -> T_est 2/1, "State "/1
  State update/4(cov_i) -> Terminator/1
  Demux/2 -> Mux/3
  Demux/1 -> Mux/2
  T_est 1/1 -> State update/3(z)
  T_est 3/1 -> Estimated State/1
  T_est 2/1 -> Demux/1
  T_est 4/1 -> Covariance/1
  statel/1 -> State update/4(p_j)

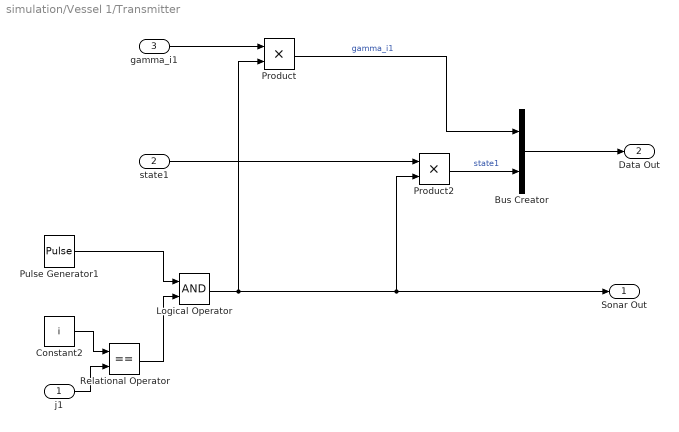
== system simulation/Vessel 1/Transmitter ==
  j1 : Inport
  state1 : Inport  Port=2
  gamma_i1 : Inport  Port=3
  Bus Creator : BusCreator  Inputs=2
  Constant2 : Constant  Value=i
  Logical Operator : Logic  AllPortsSameDT=off  OutDataTypeStr=boolean
  Product : Product
  Product2 : Product
  Pulse Generator1 : DiscretePulseGenerator  PulseType=Time based  Period=T_bc  PulseWidth=.001/( T_bc)*100
  Relational Operator : RelationalOperator  Operator===  OutDataTypeStr=boolean
  Sonar Out : Outport
  Data Out : Outport  Port=2
  wires:
  Pulse Generator1/1 -> Logical Operator/1
  j1/1 -> Relational Operator/2
  Constant2/1 -> Relational Operator/1
  Relational Operator/1 -> Logical Operator/2
  Logical Operator/1 -> Product/2, Product2/2, Sonar Out/1
  Bus Creator/1 -> Data Out/1
  gamma_i1/1 -> Product/1
  state1/1 -> Product2/1
  Product/1 -> Bus Creator/1  "gamma_i1"
  Product2/1 -> Bus Creator/2  "state1"

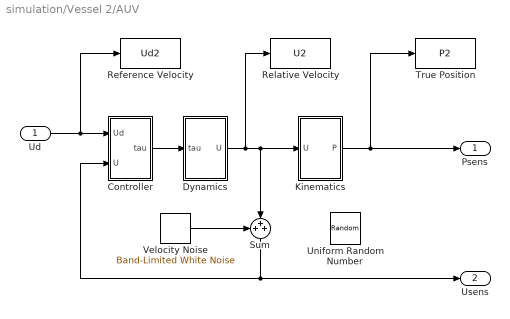
== system simulation/Vessel 2/AUV ==
  Ud : Inport
  Controller : Subsystem
  Dynamics : Subsystem
  Kinematics : Subsystem
  Reference Velocity : ToWorkspace  VariableName=Ud2  SampleTime=-1
  Relative Velocity : ToWorkspace  VariableName=U2  SampleTime=-1
  Sum : Sum  Inputs=+++
  True Position : ToWorkspace  VariableName=P2  SampleTime=-1
  Uniform Random Number : UniformRandomNumber  Minimum=-5*noiseon*[nu nv nr]  Maximum=5*noiseon*[nu nv nr]  Seed=[9274 0212 1235]  SampleTime=20
  Velocity Noise : simulink/Sources/Band-Limited White Noise  Cov=noiseon*[nu nv nr]*0.1  Ts=0.1  seed=[4729 2120 5321]
  Psens : Outport
  Usens : Outport  Port=2
  wires:
  Kinematics/1(P) -> True Position/1, Psens/1
  Sum/1 -> Usens/1, Controller/2(U)
  Velocity Noise/1 -> Sum/1
  Ud/1 -> Reference Velocity/1, Controller/1(Ud)
  Controller/1(tau) -> Dynamics/1(tau)
  Dynamics/1(U) -> Kinematics/1(U), Sum/2, Relative Velocity/1

== system simulation/Vessel 2/Compass ==
  Position : Inport
  Compass noise : simulink/Sources/Band-Limited White Noise  Cov=noiseon*npsi*0.1  Ts=0.1  seed=5246
  Demux : Demux  Outputs=3
  Mux1 : Mux  Inputs=2
  Sum : Sum  Inputs=|++
  Sum1 : Sum  Inputs=+|+
  Terminator1 : Terminator
  calibration error : simulink/Sources/Band-Limited White Noise  Cov=noiseon*npsi*200  Ts=200  seed=7425
  Psi_sens : Outport
  wires:
  Demux/2 -> Mux1/2
  Mux1/1 -> Terminator1/1
  Demux/1 -> Mux1/1
  Sum/1 -> Psi_sens/1
  Demux/3 -> Sum/1
  Position/1 -> Demux/1
  Sum1/1 -> Sum/2
  Compass noise/1 -> Sum1/1
  calibration error/1 -> Sum1/2

== system simulation/Vessel 2/Coordination State Estimator ==
  v_L : Inport
  gam_i : Inport  Port=2
  j : Inport  Port=3
  gam_j : Inport  Port=4
  Integrator2 : Integrator  InitialCondition=zeros(1,n)
  "Update " : MATLAB Function  TreatAsAtomicUnit=on
  Gam_est : Outport
  wires:
  "Update "/1(Gam_est) -> Gam_est/1
  j/1 -> "Update "/4(j)
  gam_j/1 -> "Update "/3(gam_j)
  gam_i/1 -> "Update "/2(gam_i)
  Integrator2/1 -> "Update "/1(Gam_predict)
  v_L/1 -> Integrator2/1

== system simulation/Vessel 2/Path Generator ==
  gam : Inport
  pathdata : Inport  Port=2
  id : Inport  Port=3
  Nominal Values Generator : Subsystem
  Read Pathdata : Subsystem
  Pd : Outport
  dPd : Outport  Port=2
  vL : Outport  Port=3
  wires:
  Read Pathdata/1(path params) -> Nominal Values Generator/2(path params)
  id/1 -> Read Pathdata/3(id)
  pathdata/1 -> Read Pathdata/2(pathdata)
  gam/1 -> Read Pathdata/1(gam), Nominal Values Generator/1(gam)
  Nominal Values Generator/1(P_d) -> Pd/1
  Nominal Values Generator/2(dP_d) -> dPd/1
  Nominal Values Generator/3(v_L) -> vL/1

== system simulation/Vessel 2/Path-Following Controller ==
  dgam : Inport
  P_d : Inport  Port=2
  dP_d/dgam : Inport  Port=3
  vd : Inport  Port=4
  Sensors : Inport  Port=5
  Demux : Demux  Outputs=3
  PF Control Law : MATLAB Function  TreatAsAtomicUnit=on
  Path following error : ToWorkspace  VariableName=PFerror2  SampleTime=-1
  ddgam : Outport
  U_d : Outport  Port=2
  wires:
  PF Control Law/2(e) -> Path following error/1
  Demux/2 -> PF Control Law/2(P)
  Demux/3 -> PF Control Law/3(psi)
  Demux/1 -> PF Control Law/1(Vc)
  PF Control Law/3(ddgam) -> ddgam/1
  PF Control Law/1(Ud) -> U_d/1
  dgam/1 -> PF Control Law/7(dgam)
  P_d/1 -> PF Control Law/4(Pd)
  dP_d/dgam/1 -> PF Control Law/5(dPd)
  vd/1 -> PF Control Law/6(Vd)
  Sensors/1 -> Demux/1

== system simulation/Vessel 2/Receiver ==
  Sonar In : Inport
  Data In : Inport  Port=2
  dist : Inport  Port=3
  Bus Selector : BusSelector  OutputSignals=gamma,state
  Terminator : Terminator
  state : Outport
  range_j : Outport  Port=2
  gamma_j : Outport  Port=3
  wires:
  Bus Selector/2 -> state/1  "<state>"
  Bus Selector/1 -> gamma_j/1  "<gamma>"
  dist/1 -> range_j/1
  Data In/1 -> Bus Selector/1
  Sonar In/1 -> Terminator/1

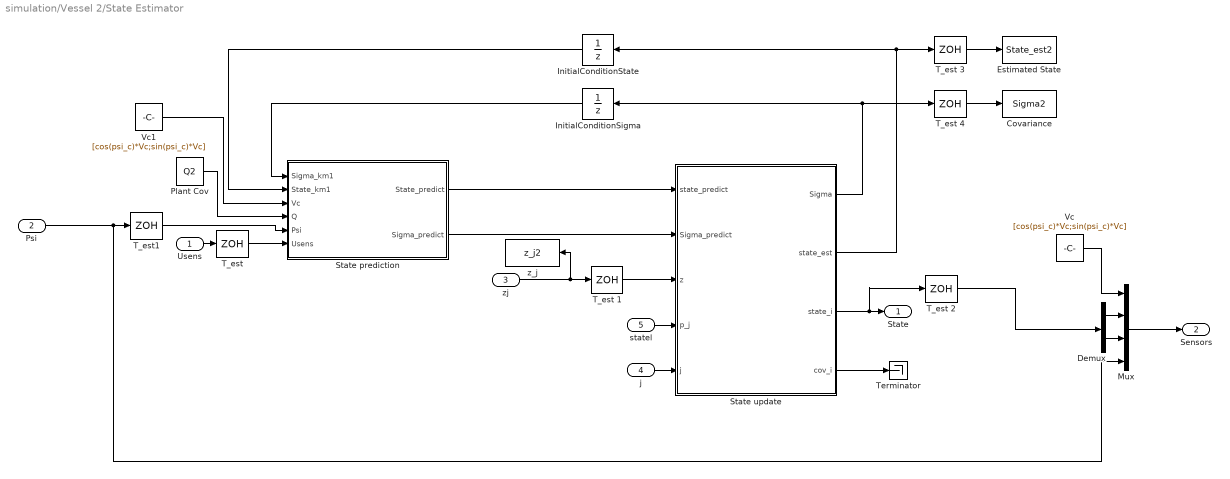
== system simulation/Vessel 2/State Estimator ==
  Usens : Inport
  Psi : Inport  Port=2
  zj : Inport  Port=3
  j : Inport  Port=4
  statel : Inport  Port=5
  Covariance : ToWorkspace  VariableName=Sigma2  SampleTime=-1
  Demux : Demux  Outputs=2
  Estimated State : ToWorkspace  VariableName=State_est2  SampleTime=-1
  InitialConditionSigma : UnitDelay  InitialCondition=Sigma02  SampleTime=T_est
  InitialConditionState : UnitDelay  InitialCondition=State_est02  SampleTime=T_est
  Mux : Mux
  Plant Cov : Constant  Value=Q2
  State prediction : MATLAB Function  TreatAsAtomicUnit=on
  State update : MATLAB Function  TreatAsAtomicUnit=on
  T_est {,1..4} (5 alike) : ZeroOrderHold  SampleTime=T_est
  "T_est1 " : ZeroOrderHold  SampleTime=T_est
  Terminator : Terminator
  Vc : Constant  Value=[cos(psi_c)*Vc;sin(psi_c)*Vc]
  Vc1 : Constant  Value=[cos(psi_c)*Vc;sin(psi_c)*Vc]
  z_j : ToWorkspace  VariableName=z_j2  SampleTime=-1
  "State " : Outport
  Sensors : Outport  Port=2
  wires:
  statel/1 -> State update/4(p_j)
  T_est 4/1 -> Covariance/1
  T_est 2/1 -> Demux/1
  T_est 3/1 -> Estimated State/1
  T_est 1/1 -> State update/3(z)
  Demux/1 -> Mux/2
  Demux/2 -> Mux/3
  State update/4(cov_i) -> Terminator/1
  State update/3(state_i) -> "State "/1, T_est 2/1
  j/1 -> State update/5(j)
  Vc1/1 -> State prediction/3(Vc)
  "T_est "/1 -> State prediction/6(Usens)
  "T_est1 "/1 -> State prediction/5(Psi)
  zj/1 -> z_j/1, T_est 1/1
  Plant Cov/1 -> State prediction/4(Q)
  Psi/1 -> "T_est1 "/1, Mux/4
  Vc/1 -> Mux/1
  Mux/1 -> Sensors/1
  Usens/1 -> "T_est "/1
  InitialConditionState/1 -> State prediction/2(State_km1)
  InitialConditionSigma/1 -> State prediction/1(Sigma_km1)
  State update/1(Sigma) -> InitialConditionSigma/1, T_est 4/1
  State prediction/2(Sigma_predict) -> State update/2(Sigma_predict)
  State update/2(state_est) -> InitialConditionState/1, T_est 3/1
  State prediction/1(State_predict) -> State update/1(state_predict)

== system simulation/Vessel 2/Transmitter ==
  j1 : Inport
  state1 : Inport  Port=2
  gamma_i1 : Inport  Port=3
  Bus Creator : BusCreator  Inputs=2
  Constant2 : Constant  Value=i
  Logical Operator : Logic  AllPortsSameDT=off  OutDataTypeStr=boolean
  Product : Product
  Product2 : Product
  Pulse Generator1 : DiscretePulseGenerator  PulseType=Time based  Period=T_bc  PulseWidth=.001/( T_bc)*100
  Relational Operator : RelationalOperator  Operator===  OutDataTypeStr=boolean
  Sonar Out : Outport
  Data Out : Outport  Port=2
  wires:
  Product2/1 -> Bus Creator/2  "state1"
  Product/1 -> Bus Creator/1  "gamma_i1"
  state1/1 -> Product2/1
  gamma_i1/1 -> Product/1
  Bus Creator/1 -> Data Out/1
  Logical Operator/1 -> Sonar Out/1, Product2/2, Product/2
  Relational Operator/1 -> Logical Operator/2
  Constant2/1 -> Relational Operator/1
  j1/1 -> Relational Operator/2
  Pulse Generator1/1 -> Logical Operator/1

== system simulation/Vessel 3/AUV ==
  Ud : Inport
  Controller : Subsystem
  Dynamics : Subsystem
  Kinematics : Subsystem
  Reference Velocity : ToWorkspace  VariableName=Ud3  SampleTime=-1
  Relative Velocity : ToWorkspace  VariableName=U3  SampleTime=-1
  Sum : Sum  Inputs=+++
  True Position : ToWorkspace  VariableName=P3  SampleTime=-1
  Uniform Random Number : UniformRandomNumber  Minimum=-5*noiseon*[nu nv nr]  Maximum=5*noiseon*[nu nv nr]  Seed=[1231 1425 5334]  SampleTime=20
  Velocity Noise : simulink/Sources/Band-Limited White Noise  Cov=noiseon*[nu nv nr]*0.1  Ts=0.1  seed=[1321 5241 4335]
  Psens : Outport
  Usens : Outport  Port=2
  wires:
  Dynamics/1(U) -> Relative Velocity/1, Sum/2, Kinematics/1(U)
  Controller/1(tau) -> Dynamics/1(tau)
  Ud/1 -> Controller/1(Ud), Reference Velocity/1
  Velocity Noise/1 -> Sum/1
  Sum/1 -> Controller/2(U), Usens/1
  Kinematics/1(P) -> Psens/1, True Position/1

== system simulation/Vessel 3/Compass ==
  Position : Inport
  Compass noise : simulink/Sources/Band-Limited White Noise  Cov=noiseon*npsi*0.1  Ts=0.1  seed=3254
  Demux : Demux  Outputs=3
  Mux1 : Mux  Inputs=2
  Sum : Sum  Inputs=|++
  Sum1 : Sum  Inputs=+|+
  Terminator1 : Terminator
  calibration error : simulink/Sources/Band-Limited White Noise  Cov=noiseon*npsi*200  Ts=200  seed=55326
  Psi_sens : Outport
  wires:
  Demux/2 -> Mux1/2
  Mux1/1 -> Terminator1/1
  Demux/1 -> Mux1/1
  Sum/1 -> Psi_sens/1
  Demux/3 -> Sum/1
  Position/1 -> Demux/1
  Sum1/1 -> Sum/2
  Compass noise/1 -> Sum1/1
  calibration error/1 -> Sum1/2

== system simulation/Vessel 3/Coordination State Estimator ==
  v_L : Inport
  gam_i : Inport  Port=2
  j : Inport  Port=3
  gam_j : Inport  Port=4
  Integrator2 : Integrator  InitialCondition=zeros(1,n)
  "Update " : MATLAB Function  TreatAsAtomicUnit=on
  Gam_est : Outport
  wires:
  v_L/1 -> Integrator2/1
  Integrator2/1 -> "Update "/1(Gam_predict)
  gam_i/1 -> "Update "/2(gam_i)
  gam_j/1 -> "Update "/3(gam_j)
  j/1 -> "Update "/4(j)
  "Update "/1(Gam_est) -> Gam_est/1

== system simulation/Vessel 3/Path Generator ==
  gam : Inport
  pathdata : Inport  Port=2
  id : Inport  Port=3
  Nominal Values Generator : Subsystem
  Read Pathdata : Subsystem
  Pd : Outport
  dPd : Outport  Port=2
  vL : Outport  Port=3
  wires:
  Nominal Values Generator/3(v_L) -> vL/1
  Nominal Values Generator/2(dP_d) -> dPd/1
  Nominal Values Generator/1(P_d) -> Pd/1
  gam/1 -> Nominal Values Generator/1(gam), Read Pathdata/1(gam)
  pathdata/1 -> Read Pathdata/2(pathdata)
  id/1 -> Read Pathdata/3(id)
  Read Pathdata/1(path params) -> Nominal Values Generator/2(path params)

== system simulation/Vessel 3/Path-Following Controller ==
  dgam : Inport
  P_d : Inport  Port=2
  dP_d/dgam : Inport  Port=3
  vd : Inport  Port=4
  Sensors : Inport  Port=5
  Demux : Demux  Outputs=3
  PF Control Law : MATLAB Function  TreatAsAtomicUnit=on
  Path following error : ToWorkspace  VariableName=PFerror3  SampleTime=-1
  ddgam : Outport
  U_d : Outport  Port=2
  wires:
  Sensors/1 -> Demux/1
  vd/1 -> PF Control Law/6(Vd)
  dP_d/dgam/1 -> PF Control Law/5(dPd)
  P_d/1 -> PF Control Law/4(Pd)
  dgam/1 -> PF Control Law/7(dgam)
  PF Control Law/1(Ud) -> U_d/1
  PF Control Law/3(ddgam) -> ddgam/1
  Demux/1 -> PF Control Law/1(Vc)
  Demux/3 -> PF Control Law/3(psi)
  Demux/2 -> PF Control Law/2(P)
  PF Control Law/2(e) -> Path following error/1

== system simulation/Vessel 3/Receiver ==
  Sonar In : Inport
  Data In : Inport  Port=2
  dist : Inport  Port=3
  Bus Selector : BusSelector  OutputSignals=gamma,state
  Terminator : Terminator
  state : Outport
  range_j : Outport  Port=2
  gamma_j : Outport  Port=3
  wires:
  Sonar In/1 -> Terminator/1
  Data In/1 -> Bus Selector/1
  dist/1 -> range_j/1
  Bus Selector/1 -> gamma_j/1  "<gamma>"
  Bus Selector/2 -> state/1  "<state>"

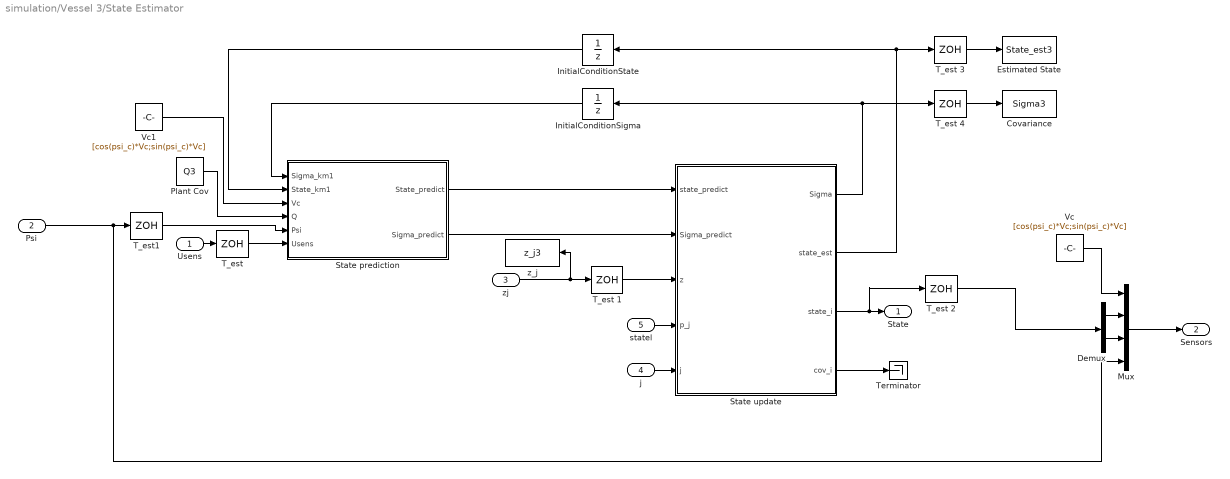
== system simulation/Vessel 3/State Estimator ==
  Usens : Inport
  Psi : Inport  Port=2
  zj : Inport  Port=3
  j : Inport  Port=4
  statel : Inport  Port=5
  Covariance : ToWorkspace  VariableName=Sigma3  SampleTime=-1
  Demux : Demux  Outputs=2
  Estimated State : ToWorkspace  VariableName=State_est3  SampleTime=-1
  InitialConditionSigma : UnitDelay  InitialCondition=Sigma03  SampleTime=T_est
  InitialConditionState : UnitDelay  InitialCondition=State_est03  SampleTime=T_est
  Mux : Mux
  Plant Cov : Constant  Value=Q3
  State prediction : MATLAB Function  TreatAsAtomicUnit=on
  State update : MATLAB Function  TreatAsAtomicUnit=on
  T_est {,1..4} (5 alike) : ZeroOrderHold  SampleTime=T_est
  "T_est1 " : ZeroOrderHold  SampleTime=T_est
  Terminator : Terminator
  Vc : Constant  Value=[cos(psi_c)*Vc;sin(psi_c)*Vc]
  Vc1 : Constant  Value=[cos(psi_c)*Vc;sin(psi_c)*Vc]
  z_j : ToWorkspace  VariableName=z_j3  SampleTime=-1
  "State " : Outport
  Sensors : Outport  Port=2
  wires:
  State prediction/1(State_predict) -> State update/1(state_predict)
  State update/2(state_est) -> T_est 3/1, InitialConditionState/1
  State prediction/2(Sigma_predict) -> State update/2(Sigma_predict)
  State update/1(Sigma) -> T_est 4/1, InitialConditionSigma/1
  InitialConditionSigma/1 -> State prediction/1(Sigma_km1)
  InitialConditionState/1 -> State prediction/2(State_km1)
  Usens/1 -> "T_est "/1
  Mux/1 -> Sensors/1
  Vc/1 -> Mux/1
  Psi/1 -> Mux/4, "T_est1 "/1
  Plant Cov/1 -> State prediction/4(Q)
  zj/1 -> T_est 1/1, z_j/1
  "T_est1 "/1 -> State prediction/5(Psi)
  "T_est "/1 -> State prediction/6(Usens)
  Vc1/1 -> State prediction/3(Vc)
  j/1 -> State update/5(j)
  State update/3(state_i) -> T_est 2/1, "State "/1
  State update/4(cov_i) -> Terminator/1
  Demux/2 -> Mux/3
  Demux/1 -> Mux/2
  T_est 1/1 -> State update/3(z)
  T_est 3/1 -> Estimated State/1
  T_est 2/1 -> Demux/1
  T_est 4/1 -> Covariance/1
  statel/1 -> State update/4(p_j)

== system simulation/Vessel 3/Transmitter ==
  j1 : Inport
  state1 : Inport  Port=2
  gamma_i1 : Inport  Port=3
  Bus Creator : BusCreator  Inputs=2
  Constant2 : Constant  Value=i
  Logical Operator : Logic  AllPortsSameDT=off  OutDataTypeStr=boolean
  Product : Product
  Product2 : Product
  Pulse Generator1 : DiscretePulseGenerator  PulseType=Time based  Period=T_bc  PulseWidth=.001/( T_bc)*100
  Relational Operator : RelationalOperator  Operator===  OutDataTypeStr=boolean
  Sonar Out : Outport
  Data Out : Outport  Port=2
  wires:
  Pulse Generator1/1 -> Logical Operator/1
  j1/1 -> Relational Operator/2
  Constant2/1 -> Relational Operator/1
  Relational Operator/1 -> Logical Operator/2
  Logical Operator/1 -> Product/2, Product2/2, Sonar Out/1
  Bus Creator/1 -> Data Out/1
  gamma_i1/1 -> Product/1
  state1/1 -> Product2/1
  Product/1 -> Bus Creator/1  "gamma_i1"
  Product2/1 -> Bus Creator/2  "state1"

== system simulation/Vessel 1/AUV/Controller ==
  Ud : Inport
  U : Inport  Port=2
  Controller : MATLAB Function  TreatAsAtomicUnit=on
  Demux : Demux  Outputs=2
  Demux1 : Demux  Outputs=3
  tau : Outport
  wires:
  Ud/1 -> Demux/1
  U/1 -> Demux1/1
  Controller/1(tau) -> tau/1
  Demux/1 -> Controller/1(ud)
  Demux/2 -> Controller/2(rd)
  Demux1/1 -> Controller/3(u)
  Demux1/2 -> Controller/4(v)
  Demux1/3 -> Controller/5(r)

== system simulation/Vessel 1/AUV/Dynamics ==
  tau : Inport
  Demux : Demux  Outputs=3
  Dynamics : MATLAB Function  TreatAsAtomicUnit=on
  Integrator : Integrator  InitialCondition=[0 0 0]
  Propellers : Subsystem
  U : Outport
  wires:
  Demux/1 -> Dynamics/1(u)
  Demux/2 -> Dynamics/2(v)
  Demux/3 -> Dynamics/3(r)
  Propellers/2(Fp) -> Dynamics/5(Fp)
  Integrator/1 -> U/1, Demux/1
  Propellers/1(Fs) -> Dynamics/4(Fs)
  tau/1 -> Propellers/1(tau)
  Dynamics/1(dU) -> Integrator/1

== system simulation/Vessel 1/AUV/Kinematics ==
  U : Inport
  Demux1 : Demux  Outputs=3
  Heading : Integrator  InitialCondition=psi01
  Kinematics : MATLAB Function  TreatAsAtomicUnit=on
  Mux : Mux  Inputs=2
  Position : Integrator  InitialCondition=P01
  Total Velocity : ToWorkspace  VariableName=Utot1  SampleTime=-1
  Vcxy : ToWorkspace  VariableName=Vcxy1  SampleTime=-1
  Water Current : Subsystem
  P : Outport
  wires:
  Kinematics/2(dP) -> Position/1
  Demux1/3 -> Heading/1
  Demux1/2 -> Kinematics/2(v)
  Demux1/1 -> Kinematics/1(u)
  U/1 -> Demux1/1
  Mux/1 -> P/1
  Position/1 -> Mux/1
  Kinematics/1(Utot) -> Total Velocity/1
  Heading/1 -> Kinematics/3(psi), Mux/2
  Water Current/1(Vcxy) -> Kinematics/4(Vc), Vcxy/1

== system simulation/Vessel 1/Path Generator/Nominal Values Generator ==
  gam : Inport
  path params : Inport  Port=2
  Bus Selector : BusSelector  OutputSignals=gamWP,thetad,P0,v_L,Circle
  MATLAB Function : MATLAB Function  TreatAsAtomicUnit=on
  P_d : Outport
  dP_d : Outport  Port=2
  v_L : Outport  Port=3
  wires:
  path params/1 -> Bus Selector/1
  MATLAB Function/1(Pd) -> P_d/1
  MATLAB Function/2(dPd) -> dP_d/1
  gam/1 -> MATLAB Function/1(gam)
  Bus Selector/1 -> MATLAB Function/2(gamWP)  "<gamWP>"
  Bus Selector/2 -> MATLAB Function/3(thetad)  "<thetad>"
  Bus Selector/3 -> MATLAB Function/4(P0)  "<P0>"
  Bus Selector/4 -> v_L/1, MATLAB Function/5(v_L)  "<v_L>"
  Bus Selector/5 -> MATLAB Function/6(Radius)  "<Circle>"

== system simulation/Vessel 1/Path Generator/Read Pathdata ==
  gam : Inport
  pathdata : Inport  Port=2
  id : Inport  Port=3
  Bus Creator : BusCreator  Inputs=5
  Path1 : MATLAB Function  TreatAsAtomicUnit=on
  path params : Outport
  wires:
  gam/1 -> Path1/2(gam)
  Path1/3(P0) -> Bus Creator/3
  Path1/1(gamWP) -> Bus Creator/1
  Path1/2(thetad) -> Bus Creator/2
  Path1/4(v_L) -> Bus Creator/4
  Bus Creator/1 -> path params/1
  pathdata/1 -> Path1/1(pathdata)
  id/1 -> Path1/3(id)
  Path1/5(Circle) -> Bus Creator/5

== system simulation/Vessel 2/AUV/Controller ==
  Ud : Inport
  U : Inport  Port=2
  Controller : MATLAB Function  TreatAsAtomicUnit=on
  Demux : Demux  Outputs=2
  Demux1 : Demux  Outputs=3
  tau : Outport
  wires:
  Demux1/3 -> Controller/5(r)
  Demux1/2 -> Controller/4(v)
  Demux1/1 -> Controller/3(u)
  Demux/2 -> Controller/2(rd)
  Demux/1 -> Controller/1(ud)
  Controller/1(tau) -> tau/1
  U/1 -> Demux1/1
  Ud/1 -> Demux/1

== system simulation/Vessel 2/AUV/Dynamics ==
  tau : Inport
  Demux : Demux  Outputs=3
  Dynamics : MATLAB Function  TreatAsAtomicUnit=on
  Integrator : Integrator  InitialCondition=[0 0 0]
  Propellers : Subsystem
  U : Outport
  wires:
  Dynamics/1(dU) -> Integrator/1
  tau/1 -> Propellers/1(tau)
  Propellers/1(Fs) -> Dynamics/4(Fs)
  Integrator/1 -> Demux/1, U/1
  Propellers/2(Fp) -> Dynamics/5(Fp)
  Demux/3 -> Dynamics/3(r)
  Demux/2 -> Dynamics/2(v)
  Demux/1 -> Dynamics/1(u)

== system simulation/Vessel 2/AUV/Kinematics ==
  U : Inport
  Demux1 : Demux  Outputs=3
  Heading : Integrator  InitialCondition=psi02
  Kinematics : MATLAB Function  TreatAsAtomicUnit=on
  Mux : Mux  Inputs=2
  Position : Integrator  InitialCondition=P02
  Total Velocity : ToWorkspace  VariableName=Utot2  SampleTime=-1
  Vcxy : ToWorkspace  VariableName=Vcxy2  SampleTime=-1
  Water Current : Subsystem
  P : Outport
  wires:
  Water Current/1(Vcxy) -> Vcxy/1, Kinematics/4(Vc)
  Heading/1 -> Mux/2, Kinematics/3(psi)
  Kinematics/1(Utot) -> Total Velocity/1
  Position/1 -> Mux/1
  Mux/1 -> P/1
  U/1 -> Demux1/1
  Demux1/1 -> Kinematics/1(u)
  Demux1/2 -> Kinematics/2(v)
  Demux1/3 -> Heading/1
  Kinematics/2(dP) -> Position/1

== system simulation/Vessel 2/Path Generator/Nominal Values Generator ==
  gam : Inport
  path params : Inport  Port=2
  Bus Selector : BusSelector  OutputSignals=gamWP,thetad,P0,v_L,Circle
  MATLAB Function : MATLAB Function  TreatAsAtomicUnit=on
  P_d : Outport
  dP_d : Outport  Port=2
  v_L : Outport  Port=3
  wires:
  Bus Selector/5 -> MATLAB Function/6(Radius)  "<Circle>"
  Bus Selector/4 -> MATLAB Function/5(v_L), v_L/1  "<v_L>"
  Bus Selector/3 -> MATLAB Function/4(P0)  "<P0>"
  Bus Selector/2 -> MATLAB Function/3(thetad)  "<thetad>"
  Bus Selector/1 -> MATLAB Function/2(gamWP)  "<gamWP>"
  gam/1 -> MATLAB Function/1(gam)
  MATLAB Function/2(dPd) -> dP_d/1
  MATLAB Function/1(Pd) -> P_d/1
  path params/1 -> Bus Selector/1

== system simulation/Vessel 2/Path Generator/Read Pathdata ==
  gam : Inport
  pathdata : Inport  Port=2
  id : Inport  Port=3
  Bus Creator : BusCreator  Inputs=5
  Path1 : MATLAB Function  TreatAsAtomicUnit=on
  path params : Outport
  wires:
  Path1/5(Circle) -> Bus Creator/5
  id/1 -> Path1/3(id)
  pathdata/1 -> Path1/1(pathdata)
  Bus Creator/1 -> path params/1
  Path1/4(v_L) -> Bus Creator/4
  Path1/2(thetad) -> Bus Creator/2
  Path1/1(gamWP) -> Bus Creator/1
  Path1/3(P0) -> Bus Creator/3
  gam/1 -> Path1/2(gam)

== system simulation/Vessel 3/AUV/Controller ==
  Ud : Inport
  U : Inport  Port=2
  Controller : MATLAB Function  TreatAsAtomicUnit=on
  Demux : Demux  Outputs=2
  Demux1 : Demux  Outputs=3
  tau : Outport
  wires:
  Ud/1 -> Demux/1
  U/1 -> Demux1/1
  Controller/1(tau) -> tau/1
  Demux/1 -> Controller/1(ud)
  Demux/2 -> Controller/2(rd)
  Demux1/1 -> Controller/3(u)
  Demux1/2 -> Controller/4(v)
  Demux1/3 -> Controller/5(r)

== system simulation/Vessel 3/AUV/Dynamics ==
  tau : Inport
  Demux : Demux  Outputs=3
  Dynamics : MATLAB Function  TreatAsAtomicUnit=on
  Integrator : Integrator  InitialCondition=[0 0 0]
  Propellers : Subsystem
  U : Outport
  wires:
  Demux/1 -> Dynamics/1(u)
  Demux/2 -> Dynamics/2(v)
  Demux/3 -> Dynamics/3(r)
  Propellers/2(Fp) -> Dynamics/5(Fp)
  Integrator/1 -> U/1, Demux/1
  Propellers/1(Fs) -> Dynamics/4(Fs)
  tau/1 -> Propellers/1(tau)
  Dynamics/1(dU) -> Integrator/1

== system simulation/Vessel 3/AUV/Kinematics ==
  U : Inport
  Demux1 : Demux  Outputs=3
  Heading : Integrator  InitialCondition=psi03
  Kinematics : MATLAB Function  TreatAsAtomicUnit=on
  Mux : Mux  Inputs=2
  Position : Integrator  InitialCondition=P03
  Total Velocity : ToWorkspace  VariableName=Utot3  SampleTime=-1
  Vcxy : ToWorkspace  VariableName=Vcxy3  SampleTime=-1
  Water Current : Subsystem
  P : Outport
  wires:
  Kinematics/2(dP) -> Position/1
  Demux1/3 -> Heading/1
  Demux1/2 -> Kinematics/2(v)
  Demux1/1 -> Kinematics/1(u)
  U/1 -> Demux1/1
  Mux/1 -> P/1
  Position/1 -> Mux/1
  Kinematics/1(Utot) -> Total Velocity/1
  Heading/1 -> Kinematics/3(psi), Mux/2
  Water Current/1(Vcxy) -> Kinematics/4(Vc), Vcxy/1

== system simulation/Vessel 3/Path Generator/Nominal Values Generator ==
  gam : Inport
  path params : Inport  Port=2
  Bus Selector : BusSelector  OutputSignals=gamWP,thetad,P0,v_L,Circle
  MATLAB Function : MATLAB Function  TreatAsAtomicUnit=on
  P_d : Outport
  dP_d : Outport  Port=2
  v_L : Outport  Port=3
  wires:
  path params/1 -> Bus Selector/1
  MATLAB Function/1(Pd) -> P_d/1
  MATLAB Function/2(dPd) -> dP_d/1
  gam/1 -> MATLAB Function/1(gam)
  Bus Selector/1 -> MATLAB Function/2(gamWP)  "<gamWP>"
  Bus Selector/2 -> MATLAB Function/3(thetad)  "<thetad>"
  Bus Selector/3 -> MATLAB Function/4(P0)  "<P0>"
  Bus Selector/4 -> v_L/1, MATLAB Function/5(v_L)  "<v_L>"
  Bus Selector/5 -> MATLAB Function/6(Radius)  "<Circle>"

== system simulation/Vessel 3/Path Generator/Read Pathdata ==
  gam : Inport
  pathdata : Inport  Port=2
  id : Inport  Port=3
  Bus Creator : BusCreator  Inputs=5
  Path1 : MATLAB Function  TreatAsAtomicUnit=on
  path params : Outport
  wires:
  gam/1 -> Path1/2(gam)
  Path1/3(P0) -> Bus Creator/3
  Path1/1(gamWP) -> Bus Creator/1
  Path1/2(thetad) -> Bus Creator/2
  Path1/4(v_L) -> Bus Creator/4
  Bus Creator/1 -> path params/1
  pathdata/1 -> Path1/1(pathdata)
  id/1 -> Path1/3(id)
  Path1/5(Circle) -> Bus Creator/5

== system simulation/Vessel 1/AUV/Dynamics/Propellers ==
  tau : Inport
  Demux1 : Demux  Outputs=2
  Fan forces : ToWorkspace  VariableName=F1  SampleTime=-1
  Gain : Gain  Gain=[.5 .5/l; .5 -.5/l]  Multiplication=Matrix(K*u)
  Saturation : Saturate  UpperLimit=Fmax  LowerLimit=Fmin
  Fs : Outport
  Fp : Outport  Port=2
  wires:
  Demux1/1 -> Fs/1
  tau/1 -> Gain/1
  Demux1/2 -> Fp/1
  Gain/1 -> Saturation/1
  Saturation/1 -> Demux1/1, Fan forces/1

== system simulation/Vessel 1/AUV/Kinematics/Water Current ==
  Sum : Sum  Inputs=++|
  Sum1 : Sum  Inputs=|++
  Vc : Constant  Value=Vc
  Vc noise : simulink/Sources/Band-Limited White Noise  Cov=nVc*5  Ts=5  seed=[23341]
  Water current : MATLAB Function  TreatAsAtomicUnit=on
  psi_c : Constant  Value=psi_c
  psi_c noise : simulink/Sources/Band-Limited White Noise  Cov=npsi_c*5  Ts=5  seed=[256]
  Vcxy : Outport
  wires:
  psi_c noise/1 -> Sum1/2
  Vc noise/1 -> Sum/1
  Water current/1(Vcxy) -> Vcxy/1
  Sum/1 -> Water current/1(Vc)
  Sum1/1 -> Water current/2(psi_c)
  Vc/1 -> Sum/2
  psi_c/1 -> Sum1/1
